simulink subsystem "txRest"  (R2022a)
settings: Solver=VariableStepAuto  StartTime=0.0  StopTime=10.0  RelTol=1e-3
values from neighbouring files (symbols this model uses):
  bitAlloc = ones(N1, 1) * bitsPerSymbol    [initSefdmModel.m]
  dataLength = codeLength * codeRate    [initSefdmModel.m]
  fecLength = 32 / parallelFactor    (= 64)    [initSefdmModel.m]
  intrlvCol = 1    [initSefdmModel.m]
  intrlvRow = parallel * 2    (= 254)    [initSefdmModel.m]
  N1 = 254    [initSefdmModel.m]
  symbolsPerFrame = bitsPerFrame / bitsPerSymbol    (= 4064)    [initSefdmModel.m]
  useInterleave = 1    [initSefdmModel.m]
libraries: commblkcod2 x1, commblkintrlv2 x1, commdigbbndam3 x1
settings Model: Creator=lsfan  LastModifiedBy=lsfan

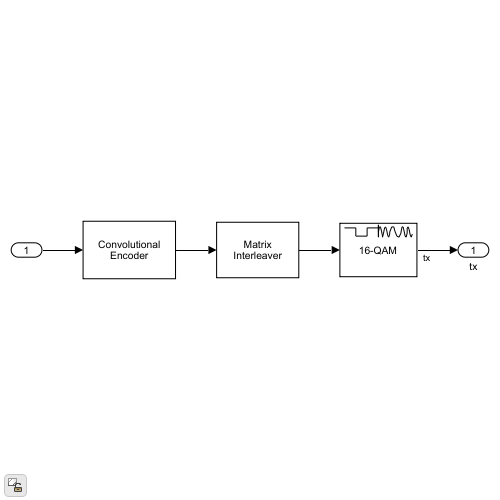
[thumbnail: Simulink's stored preview of the top-level diagram]
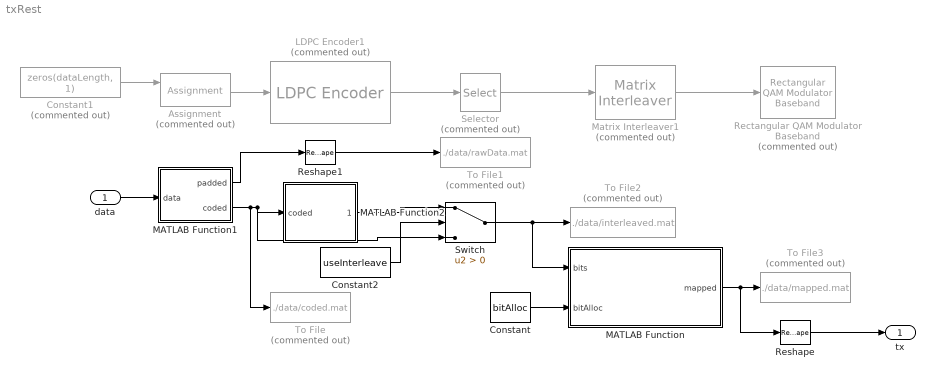
== system txRest ==
  data : Inport
  Assignment : Assignment  Commented=on  DiagnosticForDimensions=Warning  IndexOptions=Index vector (dialog)  Indices=validRange  OutputSizes=1
  Constant : Constant  Value=bitAlloc
  Constant1 : Constant  Commented=on  Value=zeros(dataLength, 1)
  Constant2 : Constant  Value=useInterleave
  LDPC Encoder1 : commblkcod2/LDPC Encoder  Commented=on  ParityCheckMat=pcmatrix
      settings: SourceProductBaseCode=CM
  MATLAB Function : MATLAB Function  TreatAsAtomicUnit=on
  MATLAB Function1 : MATLAB Function  TreatAsAtomicUnit=on
  MATLAB Function2 : MATLAB Function  TreatAsAtomicUnit=on
  Matrix Interleaver1 : commblkintrlv2/Matrix Interleaver  Commented=on  StatePerturbationForJacobian=1.0e-05  Nrows=intrlvRow  Ncols=intrlvCol
      settings: SourceProductBaseCode=CM
  Rectangular QAM Modulator Baseband : commdigbbndam3/Rectangular QAM Modulator Baseband  Commented=on  M=M  InType=Bit  Enc=Gray  Mapping=[0:15]  PowType=Average Power  MinDist=2  AvgPow=1  PeakPow=1  Ph=0  outDtype=double  outWordLen=16  outUDDataType=sfix(16)  outFracLenMode=Best precision  outFracLen=15  outDataTypeStr=double  outLastDataTypeStr=double
  Reshape : Reshape  OutputDimensionality=Customize  OutputDimensions=[N1, symbolsPerFrame / N1]
  Reshape1 : Reshape
  Selector : Selector  Commented=on  InputPortWidth=codeLength  IndexOptions=Index vector (dialog)  Indices=issuedRange  OutputSizes=1
  Switch : Switch  Criteria=u2 > Threshold  SaturateOnIntegerOverflow=off  InputSameDT=off
  To File : ToFile  Commented=on  Filename=./data/coded.mat  SaveFormat=Timeseries
  To File1 : ToFile  Commented=on  Filename=./data/rawData.mat  SaveFormat=Timeseries
  To File2 : ToFile  Commented=on  Filename=./data/interleaved.mat  SaveFormat=Timeseries
  To File3 : ToFile  Commented=on  Filename=./data/mapped.mat  SaveFormat=Timeseries
  tx : Outport
  wires:
  Constant/1 -> MATLAB Function/2(bitAlloc)
  MATLAB Function2/1(interleaved) -> Switch/1
  Constant2/1 -> Switch/2
  Matrix Interleaver1/1 -> Rectangular QAM Modulator Baseband/1
  Reshape/1 -> tx/1
  Selector/1 -> Matrix Interleaver1/1
  MATLAB Function1/1(padded) -> Reshape1/1
  Constant1/1 -> Assignment/1
  Assignment/1 -> LDPC Encoder1/1
  LDPC Encoder1/1 -> Selector/1
  Reshape1/1 -> To File1/1
  data/1 -> MATLAB Function1/1(data)
  MATLAB Function/1(mapped) -> To File3/1, Reshape/1
  MATLAB Function1/2(coded) -> To File/1, MATLAB Function2/1(coded), Switch/3
  Switch/1 -> To File2/1, MATLAB Function/1(bits)

== matlab function txRest/MATLAB Function ==
  data: bits input; mapped output; bitAlloc input; N1 parameter
function mapped = qammodFtn(bits, bitAlloc, N1)
    matrix = reshape(bits, sum(bitAlloc), []);

    temp = complex(zeros(N1, 16));
    
    current = 0;
    row = 1;
    
    for i = 1:N1
        bit = bitAlloc(i);
        slice = matrix(current + 1: current + bit, :);
        temp(row, :) = qammod(slice, 2^bit, 'InputType', 'bit', 'UnitAveragePower', 1);
        current = current + bit;
        row = row + 1;
    end

    mapped = reshape(temp, [], 1);
    
end

== matlab function txRest/MATLAB Function1 ==
  data: padded output; data input; coded output; parallel parameter; fecLength parameter
function [padded, coded] = convencFTN(data, parallel, fecLength)
    
    trellis = poly2trellis(7, [171,133]);
    data = reshape(data, parallel, fecLength-6);
    padded = [data, zeros(parallel, 6)]; % padding 0s
    
    temp = zeros(parallel,fecLength*2);
    for i = 1:parallel
        slice = padded(i, :);
        temp(i,:) = convenc(slice, trellis);
    end

    coded = reshape(temp, [], 1);
end

== matlab function txRest/MATLAB Function2 ==
  data: coded input; interleaved output; parallel parameter; intrlvCol parameter; intrlvRow parameter
function interleaved = interleave(coded, parallel, intrlvCol, intrlvRow)

    coded = reshape(coded, parallel * 2, 64);
    container = zeros(parallel * 2, 64);
    for i = 1:64
        column = coded(:,i);
        temp = matintrlv(column, intrlvRow,intrlvCol); % spatial permutation
        container(:, i) = circshift(temp, i*4); % spatial permutation by circular shift
    end

    interleaved = reshape(container, [], 1);
